simulink model "DC_Grid_Sim_Withstorage_firsttopology"  (R2022b)
settings: Solver=FixedStepAuto  StartTime=0.0  StopTime=48*4  FixedStep=0.01  RelTol=1e-3
undefined symbols (not defined in the file or in its folder): cableLV, cableMV, flexible_load_autumn_noshift, flexible_load_spring_noshift, flexible_load_summer_noshift, flexible_load_winter_noshift, LowLoadP, PeakShP, Scaling_factor, Wind_scalefactor
libraries: DC_GRIDSIM_LIB x47, simulink x8
settings Model: PauseTimes=48*2  Creator=mingreico  LastModifiedBy=mingreico

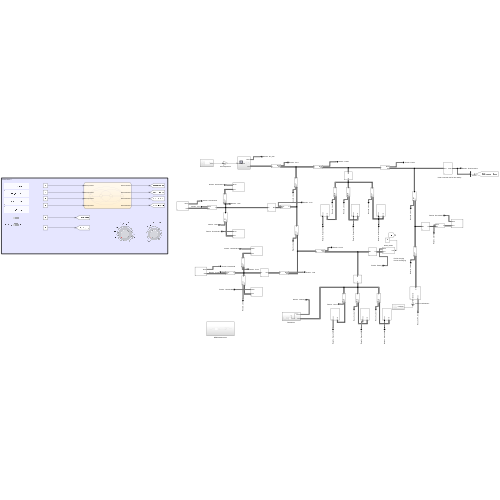
[thumbnail: Simulink's stored preview of the top-level diagram]
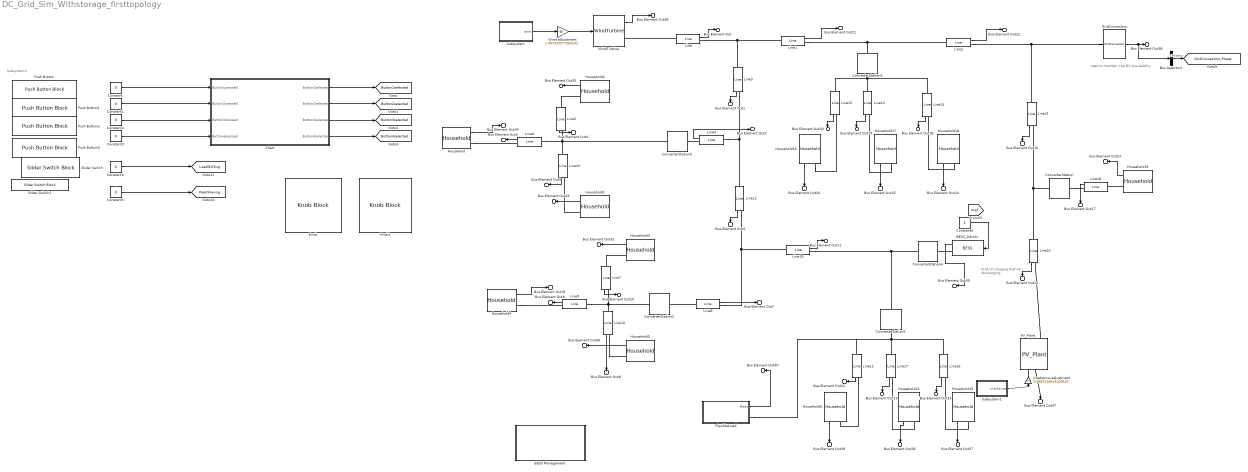
== system DC_Grid_Sim_Withstorage_firsttopology ==
  note: Pref>0 charging
      | Pref<0 discharging
  note: Subsystem1
  note: Used to maintain the DC bus stablity
  BESS Management : Subsystem
  BESS_10kAhr : DC_GRIDSIM_LIB/BESS  V_Bat=380  Qbat=10000  SOC_init=0.5  SOC_min=0.1  SOC_max=0.9  P_max=10000
      settings: SourceProductName=DC GRIDSIM Library improved
  Bus Selector2 : BusSelector  OutputSignals=Power
  Chart : Stateflow chart  TreatAsAtomicUnit=on
  Constant{,1..3} (4 alike) : Constant  Value=0  OutDataTypeStr=boolean
  Constant4 : Constant  Value=0
  Constant5 : Constant  Value=0
  Constant6 : Constant
  ConverterStation{,1..5} (6 alike) : DC_GRIDSIM_LIB/ConverterStation  V_Ref=380
      settings: SourceProductName=DC GRIDSIM Library improved
  FlexibleLoad : Subsystem
  GridConnection : DC_GRIDSIM_LIB/GridConnection  MV_Ref=MV
      settings: SourceProductName=DC GRIDSIM Library improved
  Household : DC_GRIDSIM_LIB/Household  ProfileSpring=Household15_Springallday  ProfileSummer=Household15_Summerallday  ProfileAutumn=Household15_Autumnallday  ProfileWinter=Household15_Winterallday  Timevector=Allday_timevector  k=Scaling_factor  VnomLoad=LV
      settings: SourceProductName=DC GRIDSIM Library improved
  Household1 : DC_GRIDSIM_LIB/Household  ProfileSpring=Household8_Springallday  ProfileSummer=Household8_Summerallday  ProfileAutumn=Household8_Autumnallday  ProfileWinter=Household8_Winterallday  Timevector=Allday_timevector  k=Scaling_factor  VnomLoad=LV
      settings: SourceProductName=DC GRIDSIM Library improved
  Household14 : DC_GRIDSIM_LIB/Household  ProfileSpring=Household9_Springallday  ProfileSummer=Household9_Summerallday  ProfileAutumn=Household9_Autumnallday  ProfileWinter=Household9_Winterallday  Timevector=Allday_timevector  k=Scaling_factor  VnomLoad=LV
      settings: SourceProductName=DC GRIDSIM Library improved
  Household15 : DC_GRIDSIM_LIB/Household  ProfileSpring=Household10_Springallday  ProfileSummer=Household10_Summerallday  ProfileAutumn=Household10_Autumnallday  ProfileWinter=Household10_Winterallday  Timevector=Allday_timevector  k=Scaling_factor  VnomLoad=LV
      settings: SourceProductName=DC GRIDSIM Library improved
  Household16 : DC_GRIDSIM_LIB/Household  ProfileSpring=Household11_Springallday  ProfileSummer=Household11_Summerallday  ProfileAutumn=Household11_Autumnallday  ProfileWinter=Household11_Winterallday  Timevector=Allday_timevector  k=Scaling_factor  VnomLoad=LV
      settings: SourceProductName=DC GRIDSIM Library improved
  Household17 : DC_GRIDSIM_LIB/Household  ProfileSpring=Household7_Springallday  ProfileSummer=Household7_Summerallday  ProfileAutumn=Household7_Autumnallday  ProfileWinter=Household7_Winterallday  Timevector=Allday_timevector  k=Scaling_factor  VnomLoad=LV
      settings: SourceProductName=DC GRIDSIM Library improved
  Household18 : DC_GRIDSIM_LIB/Household  ProfileSpring=Household12_Springallday  ProfileSummer=Household12_Summerallday  ProfileAutumn=Household12_Autumnallday  ProfileWinter=Household12_Winterallday  Timevector=Allday_timevector  k=Scaling_factor  VnomLoad=LV
      settings: SourceProductName=DC GRIDSIM Library improved
  Household19 : DC_GRIDSIM_LIB/Household  ProfileSpring=Household14_Springallday  ProfileSummer=Household14_Summerallday  ProfileAutumn=Household14_Autumnallday  ProfileWinter=Household14_Winterallday  Timevector=Allday_timevector  k=Scaling_factor  VnomLoad=LV
      settings: SourceProductName=DC GRIDSIM Library improved
  Household2 : DC_GRIDSIM_LIB/Household  ProfileSpring=Household3_Springallday  ProfileSummer=Household3_Summerallday  ProfileAutumn=Household3_Autumnallday  ProfileWinter=Household3_Winterallday  Timevector=Allday_timevector  k=Scaling_factor  VnomLoad=LV
      settings: SourceProductName=DC GRIDSIM Library improved
  Household3 : DC_GRIDSIM_LIB/Household  ProfileSpring=Household4_Springallday  ProfileSummer=Household4_Summerallday  ProfileAutumn=Household4_Autumnallday  ProfileWinter=Household4_Winterallday  Timevector=Allday_timevector  k=Scaling_factor  VnomLoad=LV
      settings: SourceProductName=DC GRIDSIM Library improved
  Household4 : DC_GRIDSIM_LIB/Household  ProfileSpring=Household26_Springallday  ProfileSummer=Household26_Summerallday  ProfileAutumn=Household26_Autumnallday  ProfileWinter=Household26_Winterallday  Timevector=Allday_timevector  k=Scaling_factor  VnomLoad=LV
      settings: SourceProductName=DC GRIDSIM Library improved
  Household5 : DC_GRIDSIM_LIB/Household  ProfileSpring=Household9_Springallday  ProfileSummer=Household9_Summerallday  ProfileAutumn=Household9_Autumnallday  ProfileWinter=Household9_Winterallday  Timevector=Allday_timevector  k=Scaling_factor  VnomLoad=LV
      settings: SourceProductName=DC GRIDSIM Library improved
  Household6 : DC_GRIDSIM_LIB/Household  ProfileSpring=Household33_Springallday  ProfileSummer=Household33_Summerallday  ProfileAutumn=Household33_Autumnallday  ProfileWinter=Household33_Winterallday  Timevector=Allday_timevector  k=Scaling_factor  VnomLoad=LV
      settings: SourceProductName=DC GRIDSIM Library improved
  "Irradiance-adjustment " : Gain  Gain=0.9883216814160616
  Knob : KnobBlock  ScaleMin=0.9  ScaleMax=3  TickInterval=0.1
  Knob1 : KnobBlock  ScaleMin=0.9  ScaleMax=3  TickInterval=0.1
  Line{,1..4,8,12,19,21..22} (10 alike) : DC_GRIDSIM_LIB/Line  rho=rhoCopper  l=2.0  A=cableMV
      settings: SourceProductName=DC GRIDSIM Library improved
  Line{5..7,9..11,13..18,23} (13 alike) : DC_GRIDSIM_LIB/Line  rho=rhoCopper  l=2.0  A=cableLV
      settings: SourceProductName=DC GRIDSIM Library improved
  PV_Plant : DC_GRIDSIM_LIB/PV_Plant  eta_pv=0.2  area_pv=1000
      settings: SourceProductName=DC GRIDSIM Library improved
  Push Button : PushButtonBlock  ButtonText=Button_SpringAllday  OffValue=0.000000
  Push Button1 : PushButtonBlock  ButtonText=Button_SummerAllday  OffValue=0.000000
  Push Button2 : PushButtonBlock  ButtonText=Button_AutumnAllday  OffValue=0.000000
  Push Button3 : PushButtonBlock  ButtonText=Button_WinterAllday  OffValue=0.000000
  Slider Switch : SliderSwitchBlock  LabelPosition=Hide
      settings: Values={{'NOShift', 'FlexibleLoad_Shifted'}, [0 1]}
  Slider Switch1 : SliderSwitchBlock  LabelPosition=Hide
      settings: Values={{'NoPeakShaving', 'Peakshaved'}, [0 1]}
  Subsystem : Subsystem
  Subsystem1 : Subsystem
  Wind-adjustment : Gain  Gain=1.007345577569242
  WindTurbine : DC_GRIDSIM_LIB/WindTurbine  SystemSampleTime=-1  VariantActivationTime=update diagram  Latency=0  AutoFrameSizeCalculation=off
      link override Blade radius: Value=24
      settings: SourceProductName=DC GRIDSIM Library improved
  Bus Element Out : Outport  PortName=Results  Element=Line1
  Bus Element Out1 : Outport  PortName=Results  Element=Line2
  Bus Element Out2 : Outport  PortName=Results  Element=Line3
  Bus Element Out3 : Outport  PortName=Results  Element=Line4
  Bus Element Out4 : Outport  PortName=Results  Element=Line5
  Bus Element Out5 : Outport  PortName=Results  Element=Line6
  Bus Element Out6 : Outport  PortName=Results  Element=Line7
  Bus Element Out7 : Outport  PortName=Results  Element=Line8
  Bus Element Out8 : Outport  PortName=Results  Element=Line9
  Bus Element Out9 : Outport  PortName=Results  Element=Line10
  Bus Element Out10 : Outport  PortName=Results  Element=Line11
  Bus Element Out11 : Outport  PortName=Results  Element=Line12
  Bus Element Out12 : Outport  PortName=Results  Element=Line13
  Bus Element Out13 : Outport  PortName=Results  Element=Line14
  Bus Element Out14 : Outport  PortName=Results  Element=Line15
  Bus Element Out15 : Outport  PortName=Results  Element=Line16
  Bus Element Out16 : Outport  PortName=Results  Element=Line17
  Bus Element Out17 : Outport  PortName=Results  Element=Line18
  Bus Element Out18 : Outport  PortName=Results  Element=Line19
  Bus Element Out19 : Outport  PortName=Results  Element=Line20
  Bus Element Out20 : Outport  PortName=Results  Element=Line21
  Bus Element Out21 : Outport  PortName=Results  Element=Line22
  Bus Element Out22 : Outport  PortName=Results  Element=Line23
  Bus Element Out23 : Outport  PortName=Results  Element=Household1
  Bus Element Out24 : Outport  PortName=Results  Element=Household2
  Bus Element Out25 : Outport  PortName=Results  Element=Household3
  Bus Element Out26 : Outport  PortName=Results  Element=Household4
  Bus Element Out27 : Outport  PortName=Results  Element=Household5
  Bus Element Out28 : Outport  PortName=Results  Element=Household6
  Bus Element Out29 : Outport  PortName=Results  Element=Household7
  Bus Element Out30 : Outport  PortName=Results  Element=Household8
  Bus Element Out31 : Outport  PortName=Results  Element=Household9
  Bus Element Out32 : Outport  PortName=Results  Element=Household10
  Bus Element Out33 : Outport  PortName=Results  Element=Household11
  Bus Element Out34 : Outport  PortName=Results  Element=Household12
  Bus Element Out35 : Outport  PortName=Results  Element=Household13
  Bus Element Out36 : Outport  PortName=Results  Element=WT_Gen
  Bus Element Out37 : Outport  PortName=Results  Element=PV_Gen
  Bus Element Out38 : Outport  PortName=Results  Element=GridConnection
  Bus Element Out39 : Outport  PortName=Results  Element=Battery
  Bus Element Out40 : Outport  PortName=Results  Element=Flexibility
  tag scope: Button1selected=global, Button2selected=global, Button3selected=global, Button4selected=global, GridConnection_Power=global, LoadShifting=global, PeakShaving=global
  wires:
  Constant3/1 -> Chart/4(Button4pressed)
  Constant2/1 -> Chart/3(Button3pressed)
  Constant1/1 -> Chart/2(Button2pressed)
  Constant/1 -> Chart/1(Button1pressed)
  Chart/4(" Button4selected") -> [Button4selected]
  Chart/3(" Button3selected") -> [Button3selected]
  Chart/2(" Button2selected") -> [Button2selected]
  Chart/1(" Button1selected") -> [Button1selected]
  Subsystem1/1(irradiance) -> "Irradiance-adjustment "/1
  Subsystem/1(wind) -> Wind-adjustment/1
  WindTurbine/1 -> Bus Element Out36/1
  Household5/1 -> Bus Element Out30/1
  Household19/1 -> Bus Element Out23/1
  Household18/1 -> Bus Element Out24/1
  Household17/1 -> Bus Element Out25/1
  Line3/1 -> Bus Element Out1/1
  Line/1 -> Bus Element Out/1
  Line4/1 -> Bus Element Out2/1
  Line12/1 -> Bus Element Out3/1
  Line5/1 -> Bus Element Out4/1
  Line23/1 -> Bus Element Out5/1
  Line6/1 -> Bus Element Out6/1
  Line8/1 -> Bus Element Out7/1
  Line10/1 -> Bus Element Out8/1
  Line9/1 -> Bus Element Out9/1
  Line7/1 -> Bus Element Out10/1
  Line19/1 -> Bus Element Out11/1
  Line11/1 -> Bus Element Out12/1
  Line17/1 -> Bus Element Out13/1
  Line16/1 -> Bus Element Out14/1
  Line22/1 -> Bus Element Out15/1
  Line21/1 -> Bus Element Out16/1
  Line18/1 -> Bus Element Out17/1
  Line13/1 -> Bus Element Out18/1
  Line15/1 -> Bus Element Out20/1
  Line14/1 -> Bus Element Out19/1
  Line1/1 -> Bus Element Out21/1
  Line2/1 -> Bus Element Out22/1
  Household16/1 -> Bus Element Out26/1
  Household15/1 -> Bus Element Out27/1
  Household14/1 -> Bus Element Out28/1
  Household6/1 -> Bus Element Out29/1
  Household4/1 -> Bus Element Out31/1
  Household3/1 -> Bus Element Out32/1
  Household1/1 -> Bus Element Out33/1
  Household/1 -> Bus Element Out34/1
  Household2/1 -> Bus Element Out35/1
  PV_Plant/1 -> Bus Element Out37/1
  GridConnection/1 -> Bus Selector2/1, Bus Element Out38/1
  Bus Selector2/1 -> [GridConnection_Power]  "<Power>"
  Wind-adjustment/1 -> WindTurbine/1
  "Irradiance-adjustment "/1 -> PV_Plant/1
  BESS_10kAhr/1 -> Bus Element Out39/1
  Constant4/1 -> [LoadShifting]
  Constant5/1 -> [PeakShaving]
  FlexibleLoad/1(Meas) -> Bus Element Out40/1
  Constant6/1 -> BESS_10kAhr/1
  connections:
  Line/RConn1 -- Line3/LConn1 -- Line1/LConn1
  Household2/RConn1 -- Line5/LConn1
  ConverterStation3/LConn1 -- Line5/RConn1 -- Line6/LConn1 -- Line23/LConn1
  ConverterStation2/LConn1 -- Line10/LConn1 -- Line9/LConn1 -- Line7/RConn1
  Line10/RConn1 -- Household5/RConn1
  Household3/RConn1 -- Line7/LConn1
  Line3/RConn1 -- Line4/LConn1 -- Line12/LConn1
  Line19/LConn1 -- Line8/RConn1 -- Line12/RConn1
  Household17/RConn1 -- Line14/RConn1
  Household16/RConn1 -- Line15/RConn1
  Line13/RConn1 -- Household18/RConn1
  Line17/RConn1 -- Household14/RConn1
  Line19/RConn1 -- ConverterStation4/RConn1 -- ConverterStation1/RConn1
  Household15/RConn1 -- Line16/RConn1
  Household19/RConn1 -- Line18/LConn1
  PV_Plant/LConn1 -- Line22/RConn1
  GridConnection/LConn1 -- Line21/LConn1 -- Line2/RConn1
  ConverterStation5/LConn1 -- Line15/LConn1 -- Line14/LConn1 -- Line13/LConn1
  Line/LConn1 -- WindTurbine/RConn1
  Household/RConn1 -- Line6/RConn1
  Line11/RConn1 -- Household6/RConn1
  Household4/RConn1 -- Line9/RConn1
  ConverterStation5/RConn1 -- Line2/LConn1 -- Line1/RConn1
  Line22/LConn1 -- ConverterStation/RConn1 -- Line21/RConn1
  Line8/LConn1 -- ConverterStation2/RConn1
  Household1/RConn1 -- Line23/RConn1
  ConverterStation/LConn1 -- Line18/RConn1
  Line4/RConn1 -- ConverterStation3/RConn1
  BESS_10kAhr/RConn1 -- ConverterStation4/LConn1
  ConverterStation1/LConn1 -- FlexibleLoad/RConn1 -- Line11/LConn1 -- Line16/LConn1 -- Line17/LConn1

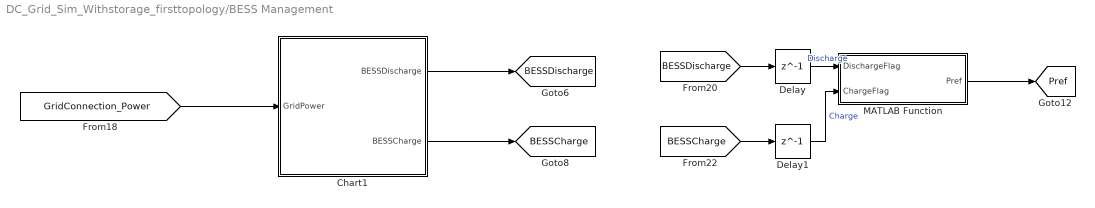
== system DC_Grid_Sim_Withstorage_firsttopology/BESS Management ==
  Chart1 : Stateflow chart  TreatAsAtomicUnit=on
  Delay : Delay  DelayLength=1
  Delay1 : Delay  DelayLength=1
  MATLAB Function : MATLAB Function  TreatAsAtomicUnit=on
  tag scope: BESSCharge=global, BESSDischarge=global, Pref=global
  wires:
  Delay1/1 -> MATLAB Function/2(ChargeFlag)  "Charge"
  Delay/1 -> MATLAB Function/1(DischargeFlag)  "Discharge"
  [BESSCharge] -> Delay1/1
  [GridConnection_Power] -> Chart1/1(GridPower)
  Chart1/1(BESSDischarge) -> [BESSDischarge]
  Chart1/2(BESSCharge) -> [BESSCharge]
  MATLAB Function/1(Pref) -> [Pref]
  [BESSDischarge] -> Delay/1

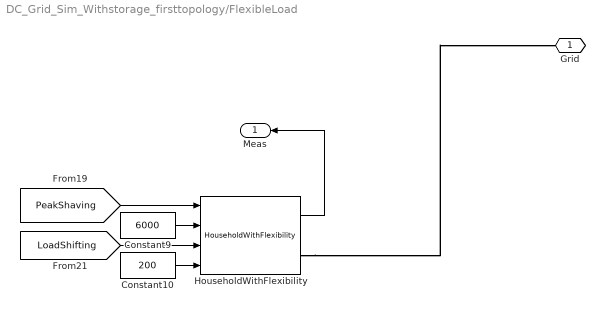
== system DC_Grid_Sim_Withstorage_firsttopology/FlexibleLoad ==
  Constant10 : Constant  Value=200
  Constant9 : Constant  Value=6000
  HouseholdWithFlexibility : DC_GRIDSIM_LIB/HouseholdWithFlexibility  Profile_spring=flexible_load_spring_noshift*10  Profile_summer=flexible_load_summer_noshift*10  Profile_autumn=flexible_load_autumn_noshift*10  Profile_winter=flexible_load_winter_noshift*10  Timevector=Allday_timevector  k=1  Vload=380  Base=800  flxQuota=0.5
      settings: SourceProductName=DC GRIDSIM Library improved
  Grid : PMIOPort  Side=Right
  Meas : Outport
  wires:
  Constant9/1 -> HouseholdWithFlexibility/2
  [LoadShifting] -> HouseholdWithFlexibility/3
  HouseholdWithFlexibility/1 -> Meas/1
  [PeakShaving] -> HouseholdWithFlexibility/1
  Constant10/1 -> HouseholdWithFlexibility/4
  connections:
  HouseholdWithFlexibility/RConn1 -- Grid/RConn1

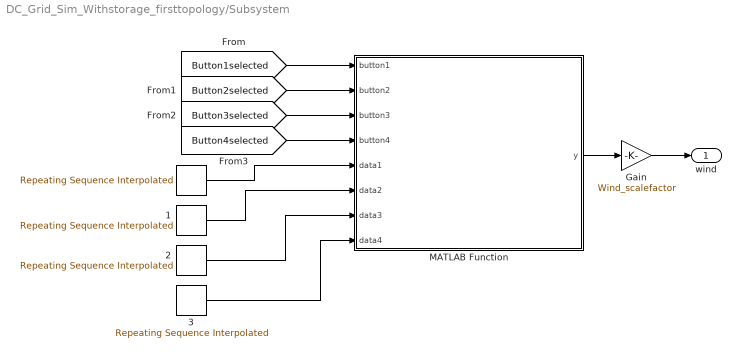
== system DC_Grid_Sim_Withstorage_firsttopology/Subsystem ==
  "  " : simulink/Sources/Repeating Sequence Interpolated  OutValues=Wind_SpringAllday  TimeValues=Allday_timevector  LookUpMeth=Interpolation-Use End Values  tsamp=0.01  OutMin=[]  OutMax=[]  OutDataTypeStr=double  OutputDataTypeScalingMode=double  OutDataType=fixdt(0,8)  OutScaling=2^-10
  "  1" : simulink/Sources/Repeating Sequence Interpolated  OutValues=Wind_SummerAllday  TimeValues=Allday_timevector  LookUpMeth=Interpolation-Use End Values  tsamp=0.01  OutMin=[]  OutMax=[]  OutDataTypeStr=double  OutputDataTypeScalingMode=double  OutDataType=fixdt(0,8)  OutScaling=2^-10
  "  2" : simulink/Sources/Repeating Sequence Interpolated  OutValues=Wind_AutumnAllday  TimeValues=Allday_timevector  LookUpMeth=Interpolation-Use End Values  tsamp=0.01  OutMin=[]  OutMax=[]  OutDataTypeStr=double  OutputDataTypeScalingMode=double  OutDataType=fixdt(0,8)  OutScaling=2^-10
  "  3" : simulink/Sources/Repeating Sequence Interpolated  OutValues=Wind_WinterAllday  TimeValues=Allday_timevector  LookUpMeth=Interpolation-Use End Values  tsamp=0.01  OutMin=[]  OutMax=[]  OutDataTypeStr=double  OutputDataTypeScalingMode=double  OutDataType=fixdt(0,8)  OutScaling=2^-10
  Gain : Gain  Gain=Wind_scalefactor
  MATLAB Function : MATLAB Function  TreatAsAtomicUnit=on
  wind : Outport
  wires:
  "  3"/1 -> MATLAB Function/8(data4)
  "  1"/1 -> MATLAB Function/6(data2)
  MATLAB Function/1(y) -> Gain/1
  "  "/1 -> MATLAB Function/5(data1)
  [Button2selected] -> MATLAB Function/2(button2)
  [Button4selected] -> MATLAB Function/4(button4)
  [Button3selected] -> MATLAB Function/3(button3)
  "  2"/1 -> MATLAB Function/7(data3)
  [Button1selected] -> MATLAB Function/1(button1)
  Gain/1 -> wind/1

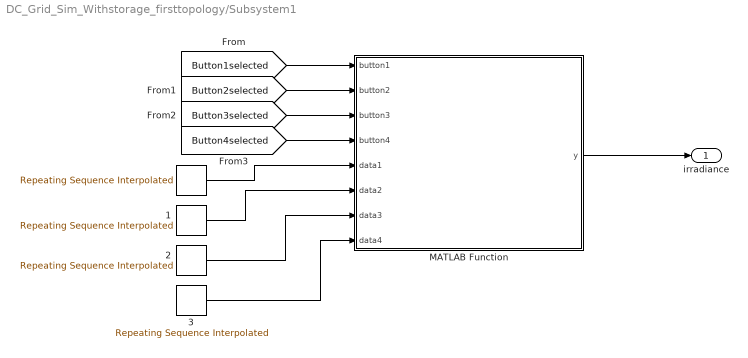
== system DC_Grid_Sim_Withstorage_firsttopology/Subsystem1 ==
  "  " : simulink/Sources/Repeating Sequence Interpolated  OutValues=Irradiance_SpringAllday  TimeValues=Allday_timevector  LookUpMeth=Interpolation-Use End Values  tsamp=0.01  OutMin=[]  OutMax=[]  OutDataTypeStr=double  OutputDataTypeScalingMode=double  OutDataType=fixdt(0,8)  OutScaling=2^-10
  "  1" : simulink/Sources/Repeating Sequence Interpolated  OutValues=Irradiance_SummerAllday  TimeValues=Allday_timevector  LookUpMeth=Interpolation-Use End Values  tsamp=0.01  OutMin=[]  OutMax=[]  OutDataTypeStr=double  OutputDataTypeScalingMode=double  OutDataType=fixdt(0,8)  OutScaling=2^-10
  "  2" : simulink/Sources/Repeating Sequence Interpolated  OutValues=Irradiance_AutumnAllday  TimeValues=Allday_timevector  LookUpMeth=Interpolation-Use End Values  tsamp=0.01  OutMin=[]  OutMax=[]  OutDataTypeStr=double  OutputDataTypeScalingMode=double  OutDataType=fixdt(0,8)  OutScaling=2^-10
  "  3" : simulink/Sources/Repeating Sequence Interpolated  OutValues=Irradiance_WinterAllday  TimeValues=Allday_timevector  LookUpMeth=Interpolation-Use End Values  tsamp=0.01  OutMin=[]  OutMax=[]  OutDataTypeStr=double  OutputDataTypeScalingMode=double  OutDataType=fixdt(0,8)  OutScaling=2^-10
  MATLAB Function : MATLAB Function  TreatAsAtomicUnit=on
  irradiance : Outport
  wires:
  "  3"/1 -> MATLAB Function/8(data4)
  "  1"/1 -> MATLAB Function/6(data2)
  [Button1selected] -> MATLAB Function/1(button1)
  "  2"/1 -> MATLAB Function/7(data3)
  [Button3selected] -> MATLAB Function/3(button3)
  [Button4selected] -> MATLAB Function/4(button4)
  [Button2selected] -> MATLAB Function/2(button2)
  "  "/1 -> MATLAB Function/5(data1)
  MATLAB Function/1(y) -> irradiance/1

== matlab function DC_Grid_Sim_Withstorage_firsttopology/Subsystem1/MATLAB Function ==
  data: button1 input; button2 input; button3 input; button4 input; data1 input; data2 input; y output; data3 input; data4 input
function y = fcn(button1, button2, button3, button4, data1,data2,data3, data4)
    if button1
        y = data1;
    elseif button2
        y =data2;
    elseif button3
        y = data3;
    elseif button4
        y = data4;
    else 
        y = data1;
    end
end

== matlab function DC_Grid_Sim_Withstorage_firsttopology/BESS Management/MATLAB Function ==
  data: DischargeFlag input; Pref output; ChargeFlag input
function Pref = fcn(DischargeFlag, ChargeFlag)
    if ChargeFlag == 1
        Pref = 10000;
    elseif DischargeFlag == 1
         Pref = -5000;
    elseif ChargeFlag == 0 && DischargeFlag == 0
        Pref = 0;
    else 
        Pref = 0;
    end

== matlab function DC_Grid_Sim_Withstorage_firsttopology/Subsystem/MATLAB Function ==
  data: button1 input; button2 input; button3 input; button4 input; data1 input; data2 input; y output; data3 input; data4 input
function y = fcn(button1, button2, button3, button4, data1,data2,data3, data4)
    if button1
        y = data1;
    elseif button2
        y =data2;
    elseif button3
        y = data3;
    elseif button4
        y = data4;
    else 
        y = data1;
    end
end

== stateflow chart DC_Grid_Sim_Withstorage_firsttopology/BESS Management/Chart1 ==
  state Initial_Mode
    entry:
    BESSDischarge=0;
    BESSCharge=0;
    exit:
    BESSDischarge=0;
    BESSCharge=0;
  state Mode1_NormalLoading
    entry:
    BESSDischarge=0;
    BESSCharge=0;
    exit:
    BESSDischarge=0;
    BESSCharge=0;
  state Mode3_BESSCharging
    entry:
    BESSDischarge=0;
    BESSCharge=1;
    exit:
    BESSDischarge=0;
    BESSCharge=0;
  note: -10
  note: 4e4
  state Mode2_PeakShaving
    entry:
    BESSDischarge=1;
    BESSCharge=0;
    exit:
    BESSDischarge=0;
    BESSCharge=0;
  Mode1_NormalLoading -> Mode3_BESSCharging [order 1] : [duration (GridPower<LowLoadP)>1]
  (default) -> Initial_Mode
  Initial_Mode -> Mode1_NormalLoading : [after(1,sec)]
  Mode3_BESSCharging -> Mode1_NormalLoading : [duration (GridPower>LowLoadP)>1]
  Mode2_PeakShaving -> Mode1_NormalLoading : [duration(GridPower<PeakShP)>1]
  Mode1_NormalLoading -> Mode2_PeakShaving [order 2] : [duration (GridPower>PeakShP)>1]
  data: GridPower input; BESSDischarge output; BESSCharge output; LowLoadP parameter; PeakShP parameter

== stateflow chart DC_Grid_Sim_Withstorage_firsttopology/Chart ==
  settings: executeAtInitialization=1
  state Button1selected
  state Button2selected
  state Button3selected
  state Button4selected
  Button1selected -> Button4selected [order 4] : [Button4pressed]
  Button2selected -> Button4selected [order 4] : [Button4pressed]
  Button1selected -> Button3selected [order 3] : [Button3pressed]
  (default) -> Button1selected
  Button3selected -> Button4selected [order 2] : [Button4pressed]
  Button2selected -> Button3selected [order 2] : [Button3pressed]
  Button1selected -> Button1selected [order 2] : [Button1pressed]
  Button3selected -> Button2selected [order 1] : [Button2pressed]
  Button4selected -> Button4selected [order 2] : [Button4pressed]
  Button1selected -> Button2selected [order 1] : [Button2pressed]
  Button4selected -> Button3selected [order 1] : [Button3pressed]
  Button2selected -> Button1selected [order 1] : [Button1pressed]
  Button3selected -> Button3selected [order 3] : [Button3pressed]
  Button3selected -> Button1selected [order 4] : [Button1pressed]
  Button4selected -> Button1selected [order 3] : [Button1pressed]
  Button2selected -> Button2selected [order 3] : [Button2pressed]
  Button4selected -> Button2selected [order 4] : [Button2pressed]
  data: Button1selected output boolean; Button2selected output boolean; Button3selected output boolean; Button1pressed input boolean size=1; Button2pressed input boolean size=1; Button3pressed input boolean size=1; Button4pressed input boolean size=1; Button4selected output boolean
